simulink model "fahrg4_b"  (R2021a)
settings: Solver=ode45  StartTime=0.0  StopTime=30  FixedStep=0.01  RelTol=1e-3  AbsTol=1e-6
libraries: Regler x2
settings Model: ExtModeTrigMode=oneshot  ExtModeArmWhenConnect=off  Creator=zimmerma  LastModifiedBy=Manoli
settings SolverCC: AutoScaleAbsTol=off  AlgebraicLoopSolver=TrustRegion
settings DataIOCC: SaveFormat=Array  SignalLoggingSaveFormat=ModelDataLogs  SaveOutput=off  SaveTime=off  ReturnWorkspaceOutputs=off  SignalLoggingName=sigsOut
settings OptimizationCC: BooleanDataType=off  ExpressionDepthLimit=2147483647  InitFltsAndDblsToZero=on  LifeSpan=inf
settings DebuggingCC: SaveWithParameterizedLinksMsg=none  UnderspecifiedInitializationDetection=Classic  MergeDetectMultiDrivingBlocksExec=none  SignalResolutionControl=TryResolveAllWithWarning  MultiTaskDSMMsg=warning  MultiTaskCondExecSysMsg=none  AllowSymbolicDim=off  StateNameClashWarn=warning  SFUnexpectedBacktrackingDiag=warning  SFNoUnconditionalDefaultTransitionDiag=warning  SFExecutionAtInitializationDiag=none  SFMachineParentedDataDiag=warning  ArithmeticOperatorsInVariantConditions=warning
settings HardwareCC: ProdBitPerPointer=32  ProdBitPerSizeT=32  ProdBitPerPtrDiffT=32  ProdLargestAtomicFloat=None  ProdIntDivRoundTo=Undefined  ProdEndianess=Unspecified  ProdWordSize=32  ProdHWDeviceType=32-bit Generic  TargetUnknown=on
settings ModelReferenceCC: PropagateSignalLabelsOutOfModel=off
settings SFSimCC: SimUseLocalCustomCode=off  SimParseCustomCode=off  CustomCodeUndefinedFunction=UseInterfaceOnly
settings RTWCC: RTWUseLocalCustomCode=off
settings CodeAppCC: StateflowObjectComments=on
settings GRTTargetCC: TargetFcnLib=ansi_tfl_tmw.mat  TargetLangStandard=C89/C90 (ANSI)  ModelReferenceCompliant=off  CombineOutputUpdateFcns=off  MatFileLogging=off  GRTInterface=on
settings ConfigComp: CovMetricSettings=dw  CovSaveCumulativeToWorkspaceVar=on  CovSaveSingleToWorkspaceVar=on  CovExternalEMLEnable=off

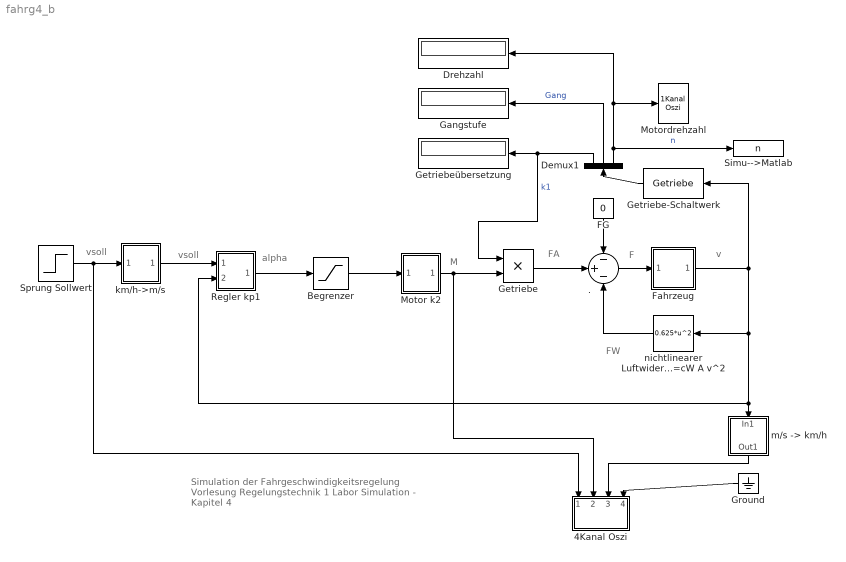
== system fahrg4_b ==
  note: Simulation der Fahrgeschwindigkeitsregelung
      | Vorlesung Regelungstechnik 1
      | Labor Simulation - Kapitel 4
  note: alpha
  note: M
  note: FA
  note: F
  note: FW
  note: v
  note: vsoll
  note: vsoll
  . : Sum  Inputs=-+-  InputSameDT=on  SaturateOnIntegerOverflow=on  OutDataTypeStr=Inherit: Same as first input
  4Kanal Oszi : Subsystem  mask(Oszilloskop){N=20000, k=[1 1 1 1], y=[-5 5], tmax=1}
      mask prompts: N "maximale Anzahl der Abtastpunkte N:"; k "Kanalverstaerkungen:"; y "[ymin ymax]:"
      mask help:
      | 4 Kanal Oszilloskop
      | Kanal1:rot    Kanal2:blau
      | Kanal3:grün Kanal4:magenta
      |
      | Achtung: Wenn das 4 Kanal Oszilloskop mehrfach in einem Blockschaltbild
      | verwendet  wird, müssen die Bezeichnungen der Variablen x1, ..., x4 und t in
      | den Simulink->Matlab Blöcken geändert werden (Edit - Look under Mask),
      | sonst überschreiben die Signale eines Oszilloskops die Werte des anderen
      | Oszilloskops im Matlab-Workspace.
      mask Help: 4 Kanal Oszilloskop mit automat. Skalierung\nKanalverstärkung einstellbar\nKanal1:rot, Kanal2:blau\nKanal3:grün, Kanal4:magenta
      mask Display: disp('Oszi')
  Begrenzer : Saturate  UpperLimit=30  LowerLimit=0
  Demux1 : Demux  Outputs=3
  Drehzahl : Display
  FG : Constant  Value=0
  Fahrzeug : Subsystem  mask(I-Glied 1/sTi mit Anfangswert u0){Ti=1600, u0=60*1000/3600}
      mask prompts: Ti "Integrationszeitkonstante Ti"; u0 "Anfangswert"
      mask help: I-Glied mit Anfangswert u0
      mask Help: Integralglied mit Anfangswert zum Zeitpunkt 0
      mask Display: disp('I\nmit u0')
  Gangstufe : Display
  Getriebe : Product  Inputs=**
  Getriebe-Schaltwerk : MATLABFcn  MATLABFcn=Getriebe  OutputDimensions=3  Output1D=off
  Getriebeübersetzung : Display
  Ground : Ground
  Motor k2 : Subsystem  mask(P){k=236/30}
      mask prompts: k "Verstärkung k"
      mask help: P-Glied k
      mask Help: P-Glied mit Verstärkung k
      mask Display: disp('P')
  Motordrehzahl : Regler/1Kanal Oszi  TR=1  ymin=0  ymax=1  npts=inf  color='r-/b-/g-/m-'
  Regler kp1 : Subsystem  mask(P-Regler){kp=30/(40*1000/3600)}
      mask help: P
      mask Help: P-Regler mit Proportionalfaktor kp
      mask Display: disp('+        \n- P')
  Simu-->Matlab : ToWorkspace  VariableName=n
      settings: MaxDataPoints=10000
  Sprung Sollwert : Step  Time=0.000001  Before=60  After=120  SampleTime=0
  km/h->m/s : Subsystem  mask(P){k=1000/3600}
      mask prompts: k "Verstärkung k"
      mask help: P-Glied k
      mask Help: P-Glied mit Verstärkung k
      mask Display: disp('P')
  "m/s -> km/h" : Subsystem  mask(P){k=3600/1000}
      mask prompts: k "Verstärkung k"
      mask help: P-Glied k
      mask Help: P-Glied mit Verstärkung k
      mask Display: disp('P')
  nichtlinearer Luftwiderstand FW=cW A v^2 : Fcn  Expr=0.625*u^2
  wires:
  Regler kp1/1(out_1) -> Begrenzer/1
  Fahrzeug/1(Ausgang) -> Getriebe-Schaltwerk/1, nichtlinearer Luftwiderstand FW=cW A v^2/1, Regler kp1/2(in_2), "m/s -> km/h"/1(In1)
  ./1 -> Fahrzeug/1(Eingang)
  Sprung Sollwert/1 -> km/h->m/s/1(In1), 4Kanal Oszi/1(in_1)
  Motor k2/1(Out1) -> Getriebe/2, 4Kanal Oszi/2(in_2)
  Getriebe/1 -> ./2
  FG/1 -> ./1
  nichtlinearer Luftwiderstand FW=cW A v^2/1 -> ./3
  km/h->m/s/1(Out1) -> Regler kp1/1(in_1)
  "m/s -> km/h"/1(Out1) -> 4Kanal Oszi/3(in_3)
  Ground/1 -> 4Kanal Oszi/4(in_4)
  Begrenzer/1 -> Motor k2/1(In1)
  Getriebe-Schaltwerk/1 -> Demux1/1
  Demux1/1 -> Getriebe/1, Getriebeübersetzung/1  "k1"
  Demux1/2 -> Gangstufe/1  "Gang"
  Demux1/3 -> Drehzahl/1, Motordrehzahl/1, Simu-->Matlab/1  "n"

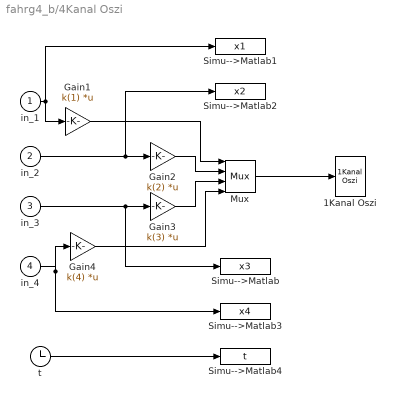
== system fahrg4_b/4Kanal Oszi ==
  in_1 : Inport
  in_2 : Inport  Port=2
  in_3 : Inport  Port=3
  in_4 : Inport  Port=4
  1Kanal Oszi : Regler/1Kanal Oszi  TR=1  ymin=0  ymax=1  npts=1024  color='r-/b-/g-/m-'
  Gain1 : Gain  Gain=k(1)  Multiplication=Matrix(K*u)  SaturateOnIntegerOverflow=on  OutDataTypeStr=Inherit: Same as input  ParamDataTypeStr=Inherit: Same as input
  Gain2 : Gain  Gain=k(2)  Multiplication=Matrix(K*u)  SaturateOnIntegerOverflow=on  OutDataTypeStr=Inherit: Same as input  ParamDataTypeStr=Inherit: Same as input
  Gain3 : Gain  Gain=k(3)  Multiplication=Matrix(K*u)  SaturateOnIntegerOverflow=on  OutDataTypeStr=Inherit: Same as input  ParamDataTypeStr=Inherit: Same as input
  Gain4 : Gain  Gain=k(4)  Multiplication=Matrix(K*u)  SaturateOnIntegerOverflow=on  OutDataTypeStr=Inherit: Same as input  ParamDataTypeStr=Inherit: Same as input
  Mux : Mux
  Simu-->Matlab : ToWorkspace  VariableName=x3
      settings: MaxDataPoints=N
  Simu-->Matlab1 : ToWorkspace  VariableName=x1
      settings: MaxDataPoints=N
  Simu-->Matlab2 : ToWorkspace  VariableName=x2
      settings: MaxDataPoints=N
  Simu-->Matlab3 : ToWorkspace  VariableName=x4
      settings: MaxDataPoints=N
  Simu-->Matlab4 : ToWorkspace  VariableName=t
      settings: MaxDataPoints=N
  t : Clock
  wires:
  t/1 -> Simu-->Matlab4/1
  Mux/1 -> 1Kanal Oszi/1
  in_2/1 -> Simu-->Matlab2/1, Gain2/1
  in_3/1 -> Simu-->Matlab/1, Gain3/1
  Gain2/1 -> Mux/2
  Gain3/1 -> Mux/3
  in_4/1 -> Simu-->Matlab3/1, Gain4/1
  Gain4/1 -> Mux/4
  Gain1/1 -> Mux/1
  in_1/1 -> Simu-->Matlab1/1, Gain1/1

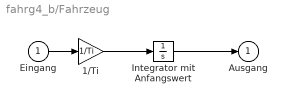
== system fahrg4_b/Fahrzeug ==
  Eingang : Inport
  "1/Ti " : Gain  Gain=1/Ti  SaturateOnIntegerOverflow=on  OutDataTypeStr=Inherit: Same as input  ParamDataTypeStr=Inherit: Same as input
  Integrator mit Anfangswert : Integrator  InitialCondition=u0
  Ausgang : Outport  VectorParamsAs1DForOutWhenUnconnected=off
  wires:
  Integrator mit Anfangswert/1 -> Ausgang/1
  Eingang/1 -> "1/Ti "/1
  "1/Ti "/1 -> Integrator mit Anfangswert/1

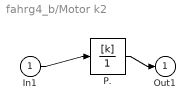
== system fahrg4_b/Motor k2 ==
  In1 : Inport
  P. : TransferFcn  Numerator=[k]  Denominator=[1]
  Out1 : Outport  VectorParamsAs1DForOutWhenUnconnected=off
  wires:
  P./1 -> Out1/1
  In1/1 -> P./1

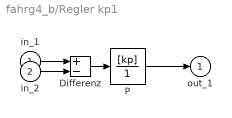
== system fahrg4_b/Regler kp1 ==
  in_1 : Inport
  in_2 : Inport  Port=2
  Differenz : Sum  Inputs=+-  InputSameDT=on  SaturateOnIntegerOverflow=on  OutDataTypeStr=Inherit: Same as first input
  P : TransferFcn  Numerator=[kp]  Denominator=[1]
  out_1 : Outport  VectorParamsAs1DForOutWhenUnconnected=off
  wires:
  in_2/1 -> Differenz/2
  in_1/1 -> Differenz/1
  P/1 -> out_1/1
  Differenz/1 -> P/1

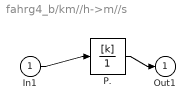
== system fahrg4_b/km//h->m//s ==
  In1 : Inport
  P. : TransferFcn  Numerator=[k]  Denominator=[1]
  Out1 : Outport  VectorParamsAs1DForOutWhenUnconnected=off
  wires:
  In1/1 -> P./1
  P./1 -> Out1/1

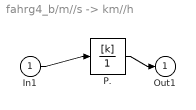
== system fahrg4_b/m//s -> km//h ==
  In1 : Inport
  P. : TransferFcn  Numerator=[k]  Denominator=[1]
  Out1 : Outport  VectorParamsAs1DForOutWhenUnconnected=off
  wires:
  In1/1 -> P./1
  P./1 -> Out1/1
